simulink model "Courant_BO"  (R2023a)
settings: Solver=VariableStepAuto  StartTime=0.0  StopTime=0.4  RelTol=1e-3
values from neighbouring files (symbols this model uses):
  Cfs = 0.350*Kc    (= 0.018375)    [parametres.m]
  f = 0    [parametres.m]
  Jm = 69.6e-3*1e-4    (= 6.96e-06)    [parametres.m]
  Jv = 10.8*Lv*1e-6    (= 3.24e-06)    [parametres.m]
  K_codeur = 23    [parametres.m]
  K_meca = 0.01    [parametres.m]
  Kc = 52.5e-3    (= 0.0525)    [parametres.m]
  Ke = 1/(182*2*pi/60)    (= 0.0524686625578)    [parametres.m]
  KI_i = 200    [parametres.m]
  KP_i = 800    [parametres.m]
  Lm = 0.62e-3    (= 0.00062)    [parametres.m]
  Rm = 2.07    [parametres.m]
  t_acc = theta_p / theta_pp    (= 0.277777777778)    [parametres.m]
  theta_p = 2.5    [parametres.m]
  Umax = 24    [parametres.m]
libraries: simulink x4
settings Model: Creator=xpess  LastModifiedBy=xpess

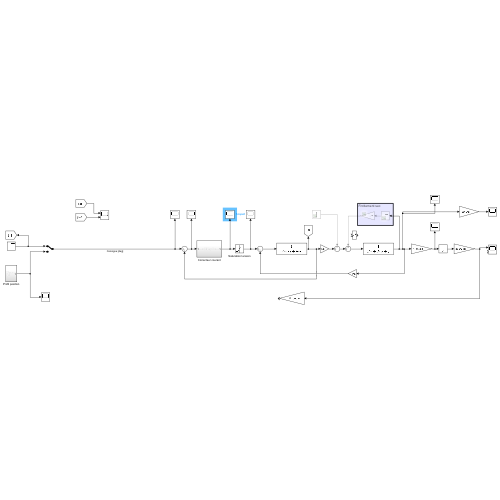
[thumbnail: Simulink's stored preview of the top-level diagram]
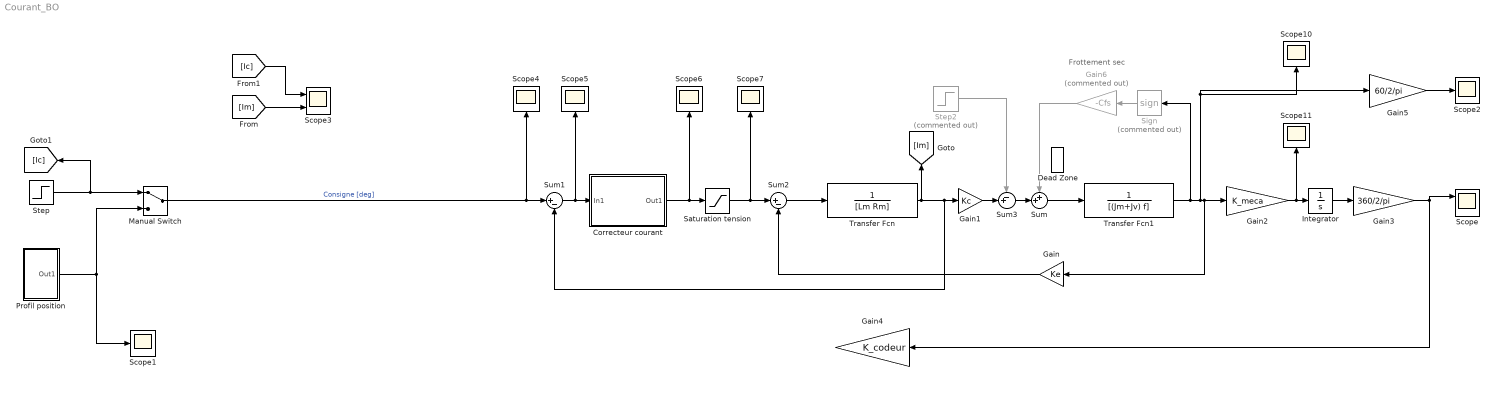
== system Courant_BO ==
  note: Frottement sec
  Correcteur courant : Subsystem
  Dead Zone : DeadZone  LowerValue=-Cfs  UpperValue=Cfs
  Gain : Gain  Gain=Ke
  Gain1 : Gain  Gain=Kc
  Gain2 : Gain  Gain=K_meca
  Gain3 : Gain  Gain=360/2/pi
  Gain4 : Gain  Gain=K_codeur
  Gain5 : Gain  Gain=60/2/pi
  Gain6 : Gain  Commented=on  Gain=-Cfs
  Integrator : Integrator
  Manual Switch : ManualSwitch
  Profil position : Subsystem
  Saturation tension : Saturate  UpperLimit=Umax  LowerLimit=-Umax
  Scope : Scope  NumInputPorts=2
  Scope{1..2,4..7,10..11} (8 alike) : Scope
  Scope3 : Scope  NumInputPorts=2
  Sign : Signum  Commented=on  ZeroCross=off
  Step : Step  Time=0.03  SampleTime=0
  Step2 : Step  Commented=on  After=0  SampleTime=0
  Sum : Sum  Inputs=++|
  Sum1 : Sum  Inputs=|+-
  Sum2 : Sum  Inputs=|+-
  Sum3 : Sum  Inputs=-+|
  Transfer Fcn : TransferFcn  Denominator=[Lm Rm]
  Transfer Fcn1 : TransferFcn  Denominator=[(Jm+Jv) f]
  wires:
  Step/1 -> [Ic], Manual Switch/1
  Transfer Fcn/1 -> Gain1/1, Sum1/2, [Im]
  Gain2/1 -> Scope11/1, Integrator/1
  Gain3/1 -> Scope/1, Gain4/1
  Manual Switch/1 -> Scope4/1, Sum1/1  "Consigne [deg]"
  Gain1/1 -> Sum3/2
  Integrator/1 -> Gain3/1
  Gain/1 -> Sum2/2
  Sum1/1 -> Scope5/1, Correcteur courant/1(In1)
  Correcteur courant/1(Out1) -> Scope6/1, Saturation tension/1
  Profil position/1(Out1) -> Manual Switch/2, Scope1/1
  Sum2/1 -> Transfer Fcn/1
  Saturation tension/1 -> Sum2/1, Scope7/1
  Gain6/1 -> Sum/1
  Transfer Fcn1/1 -> Gain5/1, Scope10/1, Gain/1, Gain2/1, Sign/1
  Sign/1 -> Gain6/1
  Sum3/1 -> Sum/2
  Step2/1 -> Sum3/1
  Sum/1 -> Transfer Fcn1/1
  Gain5/1 -> Scope2/1
  [Im] -> Scope3/2
  [Ic] -> Scope3/1

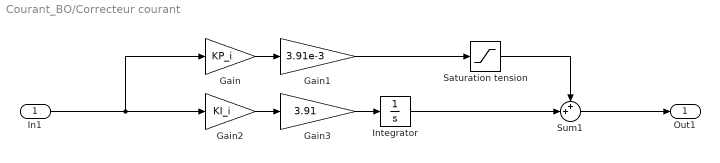
== system Courant_BO/Correcteur courant ==
  In1 : Inport
  Gain : Gain  Gain=KP_i
  Gain1 : Gain  Gain=3.91e-3
  Gain2 : Gain  Gain=KI_i
  Gain3 : Gain  Gain=3.91
  Integrator : Integrator
  Saturation tension : Saturate  UpperLimit=Umax  LowerLimit=-Umax
  Sum1 : Sum  Inputs=++|
  Out1 : Outport
  wires:
  Sum1/1 -> Out1/1
  Gain3/1 -> Integrator/1
  Integrator/1 -> Sum1/2
  Gain2/1 -> Gain3/1
  In1/1 -> Gain2/1, Gain/1
  Gain/1 -> Gain1/1
  Gain1/1 -> Saturation tension/1
  Saturation tension/1 -> Sum1/1

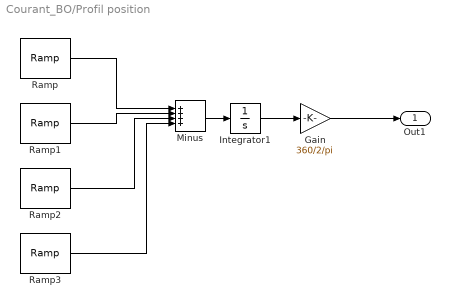
== system Courant_BO/Profil position ==
  Gain : Gain  Gain=360/2/pi
  Integrator1 : Integrator
  Minus : Sum  Inputs=++++
  Ramp : simulink/Sources/Ramp  slope=theta_p/t_acc  start=t0  InitialOutput=0
  Ramp1 : simulink/Sources/Ramp  slope=-theta_p/t_acc  start=t1  InitialOutput=0
  Ramp2 : simulink/Sources/Ramp  slope=-theta_p/t_acc  start=t2  InitialOutput=0
  Ramp3 : simulink/Sources/Ramp  slope=theta_p/t_acc  start=t3  InitialOutput=0
  Out1 : Outport
  wires:
  Ramp/1 -> Minus/1
  Integrator1/1 -> Gain/1
  Ramp3/1 -> Minus/4
  Ramp1/1 -> Minus/2
  Ramp2/1 -> Minus/3
  Minus/1 -> Integrator1/1
  Gain/1 -> Out1/1
